simulink model "DSBSC"  (R2017b)
settings: Solver=VariableStepAuto  StartTime=0.0  StopTime=0.1  RelTol=1e-3  EnableMultiTasking=on
libraries: dspsrcs4 x4, dspfdesign x3, commchan3 x1
settings Model: Creator=tuckercreger  LastModifiedBy=bgeils
settings OptimizationCC: LifeSpan=inf
settings DebuggingCC: SFUnexpectedBacktrackingDiag=warning  SFNoUnconditionalDefaultTransitionDiag=warning  SFExecutionAtInitializationDiag=none
settings CodeAppCC: StateflowObjectComments=on
settings GRTTargetCC: TargetLangStandard=C89/C90 (ANSI)  GeneratePreprocessorConditionals=Disable all
settings ConfigComp: CovMetricSettings=dw  CovHtmlReporting=on  CovSaveCumulativeToWorkspaceVar=on  CovSaveSingleToWorkspaceVar=on  CovExternalEMLEnable=off

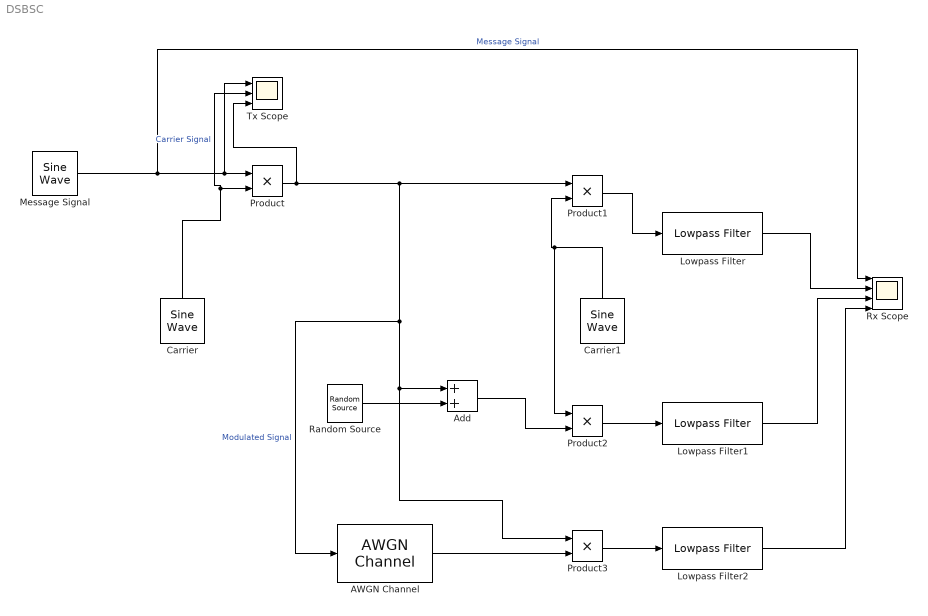
== system DSBSC ==
  AWGN Channel : commchan3/AWGN Channel  InputProcessing=Columns as channels (frame based)  seed=67  noiseMode="Signal to noise ratio  (Eb/No)"  EbNodB=10  EsNodB=10  SNRdB=10  bitsPerSym=1  Ps=1  Tsym=1  variance=1
  Add : Sum
  Carrier : dspsrcs4/Sine Wave  Amplitude=1  Frequency=1000  Phase=pi/2  SampleMode=Discrete  OutComplex=Real  CompMethod=Trigonometric fcn  TableSize=Speed  SampleTime=1/10000  SamplesPerFrame=1  ResetState=Restart at time zero  OutputFrames=off  dataType=double  wordLen=16  udDataType=sfix(16)  fracBitsMode=Best precision  numFracBits=15  OutDataTypeStr=double  LastOutDataTypeStr=double
  Carrier1 : dspsrcs4/Sine Wave  Amplitude=1  Frequency=1000  Phase=pi/2  SampleMode=Discrete  OutComplex=Real  CompMethod=Trigonometric fcn  TableSize=Speed  SampleTime=1/10000  SamplesPerFrame=1  ResetState=Restart at time zero  OutputFrames=off  dataType=double  wordLen=16  udDataType=sfix(16)  fracBitsMode=Best precision  numFracBits=15  OutDataTypeStr=double  LastOutDataTypeStr=double
  Lowpass Filter : dspfdesign/Lowpass Filter  FilterType=FIR  DesignForMinimumOrder=on  FilterOrder=50  PassbandFrequency=150  StopbandFrequency=200  PassbandRipple=0.1  StopbandAttenuation=80  InheritSampleRate=off  SampleRate=10000  SimulateUsing=Interpreted execution  roundingMode=Floor  coeffsDataTypeStr=fixdt(1,16)
  Lowpass Filter1 : dspfdesign/Lowpass Filter  FilterType=FIR  DesignForMinimumOrder=on  FilterOrder=50  PassbandFrequency=150  StopbandFrequency=200  PassbandRipple=0.1  StopbandAttenuation=80  InheritSampleRate=off  SampleRate=10000  SimulateUsing=Interpreted execution  roundingMode=Floor  coeffsDataTypeStr=fixdt(1,16)
  Lowpass Filter2 : dspfdesign/Lowpass Filter  FilterType=FIR  DesignForMinimumOrder=on  FilterOrder=50  PassbandFrequency=150  StopbandFrequency=200  PassbandRipple=0.1  StopbandAttenuation=80  InheritSampleRate=off  SampleRate=10000  SimulateUsing=Interpreted execution  roundingMode=Floor  coeffsDataTypeStr=fixdt(1,16)
  Message Signal : dspsrcs4/Sine Wave  Amplitude=1  Frequency=100  Phase=0  SampleMode=Discrete  OutComplex=Real  CompMethod=Trigonometric fcn  TableSize=Speed  SampleTime=1/10000  SamplesPerFrame=1  ResetState=Restart at time zero  OutputFrames=off  dataType=double  wordLen=16  udDataType=sfix(16)  fracBitsMode=Best precision  numFracBits=15  OutDataTypeStr=double  LastOutDataTypeStr=double
  Product{,1..3} (4 alike) : Product
  Random Source : dspsrcs4/Random Source  SrcType=Uniform  NormMethod=Ziggurat  CltLength=12  MinVal=0.5  MaxVal=1  MeanVal=0  VarVal=1  RepMode=Not repeatable  rawSeed=1  IsInherit=off  SampMode=Discrete  SampTime=10000  SampFrame=1  DataType=Single  OutComplex=Real  OutputFrames=off
  "Rx Scope " : Scope  NumInputPorts=4
  Tx Scope : Scope  NumInputPorts=3
  wires:
  Message Signal/1 -> "Rx Scope "/1, Tx Scope/1, Product/1  "Message Signal"
  Carrier/1 -> Tx Scope/2, Product/2  "Carrier Signal"
  Product/1 -> AWGN Channel/1, Add/1, Product3/1, Product1/1, Tx Scope/3  "Modulated Signal"
  Carrier1/1 -> Product2/1, Product1/2
  Product1/1 -> Lowpass Filter/1
  Random Source/1 -> Add/2
  Add/1 -> Product2/2
  Product2/1 -> Lowpass Filter1/1
  Lowpass Filter/1 -> "Rx Scope "/2
  Lowpass Filter1/1 -> "Rx Scope "/3
  AWGN Channel/1 -> Product3/2
  Product3/1 -> Lowpass Filter2/1
  Lowpass Filter2/1 -> "Rx Scope "/4
